simulink model "filter_test"  (R2018b)
settings: Solver=ode45  StartTime=0.0  StopTime=10.0  MaxStep=1e-3  RelTol=1e-4  AbsTol=1e-5
values from neighbouring files (symbols this model uses):
  xi_0 = zeros(6,1)    [RISE_params.m]
undefined symbols (not defined in the file or in its folder): ctr_params
settings Model: Creator=RUZHOU  LastModifiedBy=RUZHOU

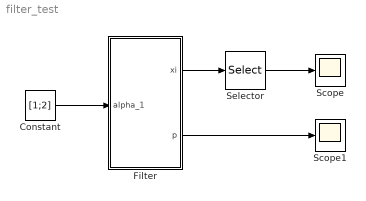
== system filter_test ==
  Constant : Constant  Value=[1;2]
  Filter : Subsystem
  Scope : Scope
  Scope1 : Scope
  Selector : Selector  InputPortWidth=6  IndexOptions=Index vector (dialog)  Indices=[1 2]  OutputSizes=1
  wires:
  Constant/1 -> Filter/1(alpha_1)
  Filter/1(xi) -> Selector/1
  Selector/1 -> Scope/1
  Filter/2(p) -> Scope1/1

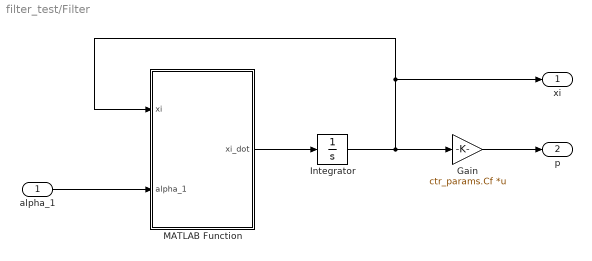
== system filter_test/Filter ==
  alpha_1 : Inport
  Gain : Gain  Gain=ctr_params.Cf  Multiplication=Matrix(K*u)
  Integrator : Integrator  InitialCondition=xi_0
  MATLAB Function : MATLAB Function  TreatAsAtomicUnit=on
  xi : Outport
  p : Outport  Port=2
  wires:
  alpha_1/1 -> MATLAB Function/2(alpha_1)
  MATLAB Function/1(xi_dot) -> Integrator/1
  Integrator/1 -> Gain/1, MATLAB Function/1(xi), xi/1
  Gain/1 -> p/1

== matlab function filter_test/Filter/MATLAB Function ==
  data: xi input size=6; xi_dot output size=6; alpha_1 input size=2; ctr_params parameter
function xi_dot = fcn(xi,alpha_1,ctr_params)
A = ctr_params.Af;
B = ctr_params.Bf;

xi_dot = A*xi + B*alpha_1;
end
